simulink model "DC_Boost_Converter"  (R2021b)
settings: Solver=ode23tb  StartTime=0.0  StopTime=0.5  MaxStep=1e-4  RelTol=1e-3
libraries: spsCurrentMeasurementLib x4, spsSeriesRLCBranchLib x3, spsDCVoltageSourceLib x1, spsDiodeLib x1, spsIGBTLib x1, spsVoltageMeasurementLib x1, spspowerguiLib x1
settings Model: Creator=90542  LastModifiedBy=90542

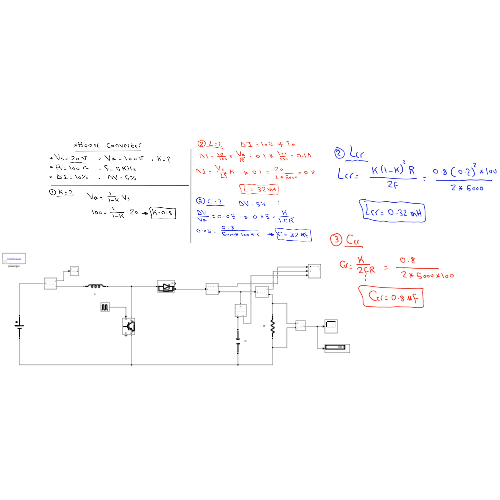
[thumbnail: Simulink's stored preview of the top-level diagram]
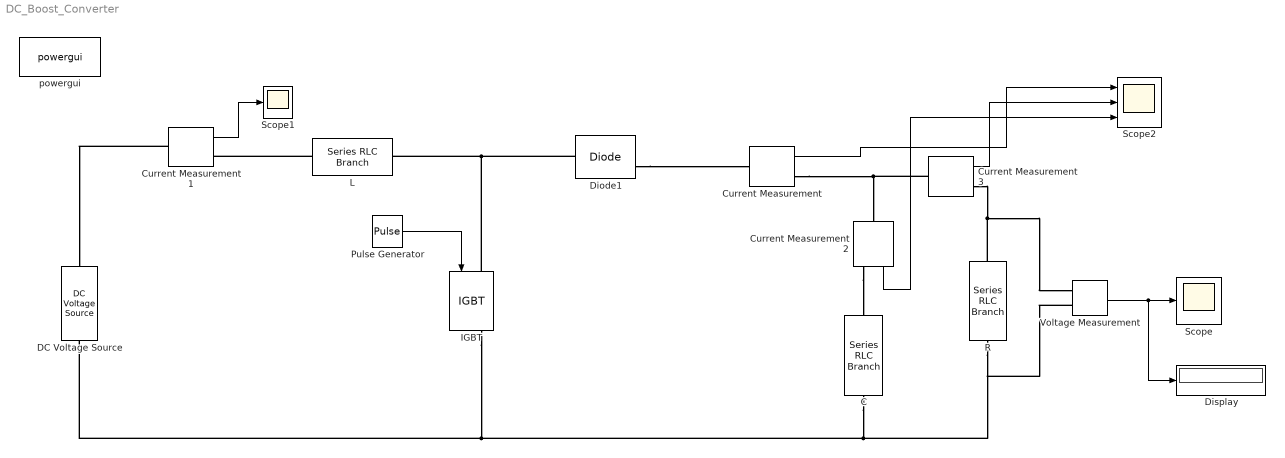
== system DC_Boost_Converter ==
  C : spsSeriesRLCBranchLib/Series RLC Branch  LConnTagsString=__new0  RConnTagsString=__new0  BranchType=C  Resistance=10  Inductance=1e-3  SetiL0=off  InitialCurrent=0  Capacitance=32e-6  Setx0=off  InitialVoltage=0  Measurements=None
  Current Measurement{,1..3} (4 alike) : spsCurrentMeasurementLib/Current Measurement  PhasorSimulation=off  OutputType=Complex  PSBequivalent=0
  DC Voltage Source : spsDCVoltageSourceLib/DC Voltage Source  Amplitude=20  Measurements=None
  Diode1 : spsDiodeLib/Diode  Ron=0.001  Lon=0  Vf=0.8  IC=0  UseSnubber=0  Rs=500  Cs=250e-9  Measurements=on
  Display : Display
  IGBT : spsIGBTLib/IGBT  Ron=0.001  Lon=0  Vf=1  Tf=1e-6  Tt=2e-6  IC=0  Rs=1e5  Cs=inf  Measurements=on
  L : spsSeriesRLCBranchLib/Series RLC Branch  LConnTagsString=__new0  RConnTagsString=__new0  BranchType=L  Resistance=10  Inductance=32e-3  SetiL0=off  InitialCurrent=0  Capacitance=1e-6  Setx0=off  InitialVoltage=0  Measurements=None
  Pulse Generator : DiscretePulseGenerator  PulseType=Time based  Period=1/5000  PulseWidth=80.5
  R : spsSeriesRLCBranchLib/Series RLC Branch  LConnTagsString=__new0  RConnTagsString=__new0  BranchType=R  Resistance=100  Inductance=1e-3  SetiL0=off  InitialCurrent=0  Capacitance=1e-6  Setx0=off  InitialVoltage=0  Measurements=None
  Scope : Scope
  Scope1 : Scope
  Scope2 : Scope  NumInputPorts=3
  Voltage Measurement : spsVoltageMeasurementLib/Voltage Measurement  PhasorSimulation=off  OutputType=Complex  PSBequivalent=0
  powergui : spspowerguiLib/powergui  Priority=1  SimulationMode=Continuous  SampleTime=50e-6  frequency=60  Iterations=50  frequencyindice=0  Pbase=100e6  ErrMax=1e-4  UnitsV=kV  UnitsW=MW  buscounter=0  FunctionMessages=off  echomessages=off  EnableUseOfTLC=off  CurrentSourceSwitches=off  DisableSnubberDevices=off  DisableRonSwitches=off  DisableVfSwitches=off  DisplayEquations=off  AutomaticDiscreteSolvers=off  SolverType=Tustin/Backward Euler (TBE)  Interpol=off  ExternalGateDelay=off  methode=off  Ts=100  x0status=blocks  SPID=on  SwTol=0  HookPort=off  NonlinearTolerance=1e-4  nMaxIteration=100  ContinueOnMaxIteration=off  RestoreLinks=warning  ResistiveCurrentMeasurement=off  Frange=[0:2:500]  Ylog=off  Xlog=on  ShowGrid=off  save=off  variable=ZData  structure=0  ZoomFFT=off  StartTime=0.0  cycles=1  DisplayStyle=1  fundamental=60  FreqAxis=off  MaxFrequency=1000  frequencyindicesteady=1  RmsSteady=1  display=off
  wires:
  Current Measurement1/1 -> Scope1/1
  Current Measurement/1 -> Scope2/1
  Voltage Measurement/1 -> Display/1, Scope/1
  Pulse Generator/1 -> IGBT/1
  Current Measurement3/1 -> Scope2/2
  Current Measurement2/1 -> Scope2/3
  connections:
  R/LConn1 -- Current Measurement3/RConn1 -- Voltage Measurement/LConn1
  L/LConn1 -- Current Measurement1/RConn1
  Current Measurement1/LConn1 -- DC Voltage Source/RConn1
  Diode1/LConn1 -- L/RConn1 -- IGBT/LConn1
  IGBT/RConn1 -- R/RConn1 -- Voltage Measurement/LConn2 -- C/LConn1 -- DC Voltage Source/LConn1
  Diode1/RConn1 -- Current Measurement/LConn1
  Current Measurement2/RConn1 -- C/RConn1
  Current Measurement/RConn1 -- Current Measurement3/LConn1 -- Current Measurement2/LConn1
